simulink model "tetherInternalForces_th"  (R2018b)
settings: Solver=VariableStepAuto  StartTime=0.0  StopTime=0  RelTol=1e-3
values from neighbouring files (symbols this model uses):
  L = 90    [tetherInternalForces_ts.m]
  N = 4    [tetherInternalForces_ts.m]
  Ri_o = [R1_o Ri_o Rn_o]    [tetherInternalForces_ts.m]
  Vi_o = zeros(size(Ri_o))    [tetherInternalForces_ts.m]
libraries: tetherInternalForces_ul x1
settings Model: Creator=asiddiq2  LastModifiedBy=asiddiq2

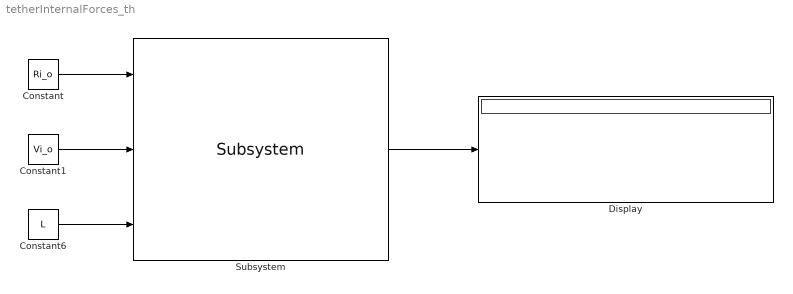
== system tetherInternalForces_th ==
  Constant : Constant  Value=Ri_o
  Constant1 : Constant  Value=Vi_o
  Constant6 : Constant  Value=L
  Display : Display
  Subsystem : tetherInternalForces_ul/Subsystem  N=N  E=E  dia_t=dia_t  mass=mass  zeta=zeta
  wires:
  Constant6/1 -> Subsystem/3
  Subsystem/1 -> Display/1
  Constant/1 -> Subsystem/1
  Constant1/1 -> Subsystem/2
